simulink library "CLICK_Lib"  (R2024b)
settings: Solver=VariableStepAuto  StartTime=0.0  StopTime=10.0  RelTol=1e-3
settings Model: Creator=pepev  LastModifiedBy=pepev

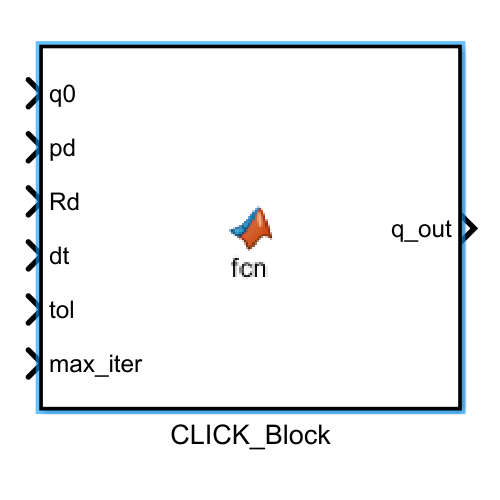
[thumbnail: Simulink's stored preview of the top-level diagram]
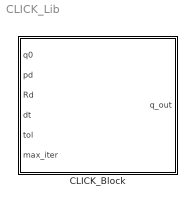
== system CLICK_Lib ==
  CLICK_Block : MATLAB Function  TreatAsAtomicUnit=on

== matlab function CLICK_Lib/CLICK_Block ==
  data: q0 input; q_out output; pd input; Rd input; dt input; tol input; max_iter input
function q_out = fcn(q0, pd, Rd, dt, tol, max_iter)
    %#codegen
    coder.extrinsic('CLICK');

    q_out = zeros(6,1); % Predefine output size for Simulink

    q_out = CLICK(q0, pd, Rd, dt, tol, max_iter);
end
